simulink model "MIL_pController"  (R2018b)
settings: Solver=FixedStepAuto  StartTime=0.0  StopTime=150  FixedStep=0.001  MaxStep=0.001  RelTol=1e-3
values from neighbouring files (symbols this model uses):
  nCyclePerMinuteRef = 25    [MIL_pController_init.m]
  Pblower_tgt = 55    [MIL_pController_init.m]
  pBlowerValveOutletMaxStaticTargetRef = 200    [MIL_pController_init.m]
  pPatientValveInletTargetRef = 100    [MIL_pController_init.m]
  rInhalationPerCycleRef = 1/3    (= 0.333333333333)    [MIL_pController_init.m]
undefined symbols (not defined in the file or in its folder): BTClockRemoval, Cpoumon, Dinttuy, e, hlibtuy, Patm, Rex, Rpoumon, sigbuilder_block, tinsp, tperiod, X_makair, Y_makair
libraries: simulink x11, simulink_extras x1
settings Model: Creator=FASSI  LastModifiedBy=VITIE
settings SolverCC: AlgebraicLoopSolver=LineSearch

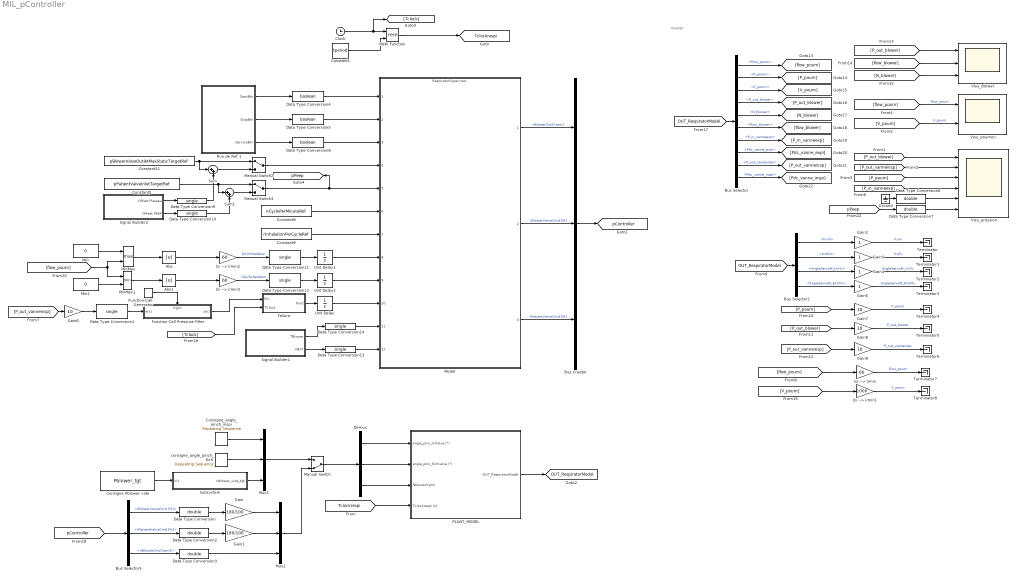
== system MIL_pController ==
  note: Viewer
  Abs : Abs
  Abs1 : Abs
  Bus Creator : BusCreator  Inputs=3
  Bus Selector : BusSelector  OutputSignals=flow_poum,P_poum,V_poum,P_out_blower,N_blower,flow_blower,P_in_vanneexp,Pdc_vanne_expi,P_out_vanneinsp,Pdc_vanne_inspi
  Bus Selector1 : BusSelector  OutputSignals=KvIn,KvExh,AngleServoM_InVlv,AngleServoM_ExhVlv
  Bus Selector5 : BusSelector  OutputSignals=rBlowerValveCmd [%],rPatientValveCmd [%],nBlowerCmd [rpm]
  Clock : Clock
  Consigne Pblower vide : Constant  Value=Pblower_tgt
  Consigne_angle_pinch_inspi : simulink/Sources/Repeating Sequence  rep_seq_t=X_insp2  rep_seq_y=[0 180 180 180 0 0 0]
  Constant1 : Constant  Value=tperiod
  Constant11 : Constant  Value=pBlowerValveOutletMaxStaticTargetRef  OutDataTypeStr=single
  Constant5 : Constant  Value=pPatientValveInletTargetRef  OutDataTypeStr=single
  Constant8 : Constant  Value=nCyclePerMinuteRef  OutDataTypeStr=single
  Constant9 : Constant  Value=rInhalationPerCycleRef  OutDataTypeStr=single
  Data Type Conversion{,2..3,6..7} (5 alike) : DataTypeConversion  OutDataTypeStr=double
  Data Type Conversion{1,9..14} (7 alike) : DataTypeConversion  OutDataTypeStr=single
  Data Type Conversion4 : DataTypeConversion  OutDataTypeStr=boolean
  Data Type Conversion5 : DataTypeConversion  OutDataTypeStr=boolean
  Data Type Conversion8 : DataTypeConversion  OutDataTypeStr=boolean
  Demux : Demux  Outputs=3
  Failure : Subsystem
  Function-Call Generator : simulink/Ports & Subsystems/Function-Call Generator  sample_time=0.005  numberOfIterations=1
  Function-Call Pressure Filter : Subsystem  TreatAsAtomicUnit=on
  Gain : Gain  Gain=180/100
  Gain1 : Gain  Gain=180/100
  Gain{2..5} (4 alike) : Gain
  Gain{6..9} (4 alike) : Gain  Gain=10
  Ground : Ground
  Manual Switch : ManualSwitch  CurrentSetting=0
  Manual Switch2 : ManualSwitch
  Manual Switch3 : ManualSwitch
  Math Function : Math  Operator=rem  SaturateOnIntegerOverflow=on
  Min : Constant  Value=0
  Min1 : Constant  Value=0
  MinMax : MinMax  Function=max  Inputs=2
  MinMax1 : MinMax  Inputs=2
  Model : ModelReference  ModelNameDialog=RespiratorSupervisor.slx  SimulationMode=Normal  ModelReferenceVersion=1.366
  Mux1 : Mux  Inputs=3
  Mux2 : Mux  Inputs=3
  PLANT_MODEL : Subsystem
  Run de Ref 1 : Subsystem  Tag=STV Subsys  LoadFcn=sigbuilder_block('load');  StartFcn=sigbuilder_block('start');  StopFcn=sigbuilder_block('stop');  ClipboardFcn=sigbuilder_block('clipboard');  mask(Sigbuilder block){tuvar=[0:10]}
      mask help: Simulink:masks:SigbuilderBlock_MD
      mask init:
      | if ~strcmp(get_param(bdroot(gcbh),'SimulationStatus'),'stopped') tuvar = sigbuilder_block('maskInit'); end
      settings: CopyFcn=sigbuilder_block('copy');  DeleteFcn=sigbuilder_block('delete');  ModelCloseFcn=sigbuilder_block('modelClose');  PreSaveFcn=sigbuilder_block('preSave');  PauseFcn=sigbuilder_block('pause');  ContinueFcn=sigbuilder_block('continue');  NameChangeFcn=sigbuilder_block('namechange');  OpenFcn=sigbuilder_block('open',[5.4 33 1141.2 514.8 ]);  CloseFcn=sigbuilder_block('close');
      mask Display: plot(0, 0, 100, 100,[2, 2, 32, 32, 2], [68, 8, 8, 68, 68],[32, 2], [38, 38], [32, 19, 2],[53, 60, 44], [32, 17, 17, 2],[16, 16, 31, 31]);txt = getActiveGroup(gcbh);text(2, 100, txt,'verticalAlignment', 'top');
  Signal Builder1 : Subsystem  Tag=STV Subsys  LoadFcn=sigbuilder_block('load');  StartFcn=sigbuilder_block('start');  StopFcn=sigbuilder_block('stop');  ClipboardFcn=sigbuilder_block('clipboard');  mask(Sigbuilder block){tuvar=[0:10]}
      mask help: Simulink:masks:SigbuilderBlock_MD
      mask init:
      | if ~strcmp(get_param(bdroot(gcbh),'SimulationStatus'),'stopped') tuvar = sigbuilder_block('maskInit'); end
      settings: CopyFcn=sigbuilder_block('copy');  DeleteFcn=sigbuilder_block('delete');  ModelCloseFcn=sigbuilder_block('modelClose');  PreSaveFcn=sigbuilder_block('preSave');  PauseFcn=sigbuilder_block('pause');  ContinueFcn=sigbuilder_block('continue');  NameChangeFcn=sigbuilder_block('namechange');  OpenFcn=sigbuilder_block('open',[5.4 30 1141.2 522.6 ]);  CloseFcn=sigbuilder_block('close');
      mask Display: plot(0, 0, 100, 100,[2, 2, 32, 32, 2], [68, 8, 8, 68, 68],[32, 2], [38, 38], [32, 19, 2],[53, 60, 44], [32, 17, 17, 2],[16, 16, 31, 31]);txt = getActiveGroup(gcbh);text(2, 100, txt,'verticalAlignment', 'top');
  Signal Builder2 : Subsystem  Tag=STV Subsys  LoadFcn=sigbuilder_block('load');  StartFcn=sigbuilder_block('start');  StopFcn=sigbuilder_block('stop');  ClipboardFcn=sigbuilder_block('clipboard');  mask(Sigbuilder block){tuvar=[0:10]}
      mask help: Simulink:masks:SigbuilderBlock_MD
      mask init:
      | if ~strcmp(get_param(bdroot(gcbh),'SimulationStatus'),'stopped') tuvar = sigbuilder_block('maskInit'); end
      settings: CopyFcn=sigbuilder_block('copy');  DeleteFcn=sigbuilder_block('delete');  ModelCloseFcn=sigbuilder_block('modelClose');  PreSaveFcn=sigbuilder_block('preSave');  PauseFcn=sigbuilder_block('pause');  ContinueFcn=sigbuilder_block('continue');  NameChangeFcn=sigbuilder_block('namechange');  OpenFcn=sigbuilder_block('open',[0 30 1152 561.6 ]);  CloseFcn=sigbuilder_block('close');
      mask Display: plot(0, 0, 100, 100,[2, 2, 32, 32, 2], [68, 8, 8, 68, 68],[32, 2], [38, 38], [32, 19, 2],[53, 60, 44], [32, 17, 17, 2],[16, 16, 31, 31]);txt = getActiveGroup(gcbh);text(2, 100, txt,'verticalAlignment', 'top');
  Subsystem : Subsystem
  Sum : Sum  Inputs=|++
  Sum1 : Sum  Inputs=|++
  Terminator{,1..8} (9 alike) : Terminator
  Unit Delay : UnitDelay  SampleTime=-1
  Unit Delay1 : UnitDelay  SampleTime=-1
  Unit Delay2 : UnitDelay  SampleTime=-1
  VIsu_Blower : Scope  NumInputPorts=3
  VIsu_poumon : Scope  NumInputPorts=2
  Visu_pression : Scope  NumInputPorts=6
  consigne_angle_pinch_Exh : simulink/Sources/Repeating Sequence  rep_seq_t=X_exp2  rep_seq_y=[0 0 0 180 180 0 0]
  l/s --> l/min : Gain  Gain=60
  l/s --> l/min1 : Gain  Gain=1000
  l/s --> l/min2 : Gain  Gain=60
  l/s --> l/min3 : Gain  Gain=60
  tag scope: OUT_RespiratorModel=global, Tclockrespi=global, pController=global, pPeep=global
  wires:
  Clock/1 -> [Tclock], Math Function/1
  Constant1/1 -> Math Function/2
  [flow_poum] -> VIsu_poumon/1  "flow_poum"
  [V_poum] -> VIsu_poumon/2  "V_poum"
  [flow_blower] -> VIsu_Blower/2
  [P_out_blower] -> VIsu_Blower/1
  [N_blower] -> VIsu_Blower/3
  Bus Selector/10 -> [Pdc_vanne_inspi]  "<Pdc_vanne_inspi>"
  Bus Selector/9 -> [P_out_vanneinsp]  "<P_out_vanneinsp>"
  Bus Selector/8 -> [Pdc_vanne_expi]  "<Pdc_vanne_expi>"
  Bus Selector/7 -> [P_in_vanneexp]  "<P_in_vanneexp>"
  Bus Selector/6 -> [flow_blower]  "<flow_blower>"
  Bus Selector/5 -> [N_blower]  "<N_blower>"
  Bus Selector/4 -> [P_out_blower]  "<P_out_blower>"
  Bus Selector/3 -> [V_poum]  "<V_poum>"
  Bus Selector/2 -> [P_poum]  "<P_poum>"
  Bus Selector/1 -> [flow_poum]  "<flow_poum>"
  [P_out_vanneinsp] -> Gain6/1
  Consigne Pblower vide/1 -> Subsystem/1(In1)
  [Tclockrespi] -> PLANT_MODEL/4(Tclockrespi (s))
  Model/3 -> Bus Creator/3  "rPatientValveCmd [%]"
  Bus Creator/1 -> [pController]
  Subsystem/1(Nblower_vide_tgt) -> Mux1/3
  consigne_angle_pinch_Exh/1 -> Mux1/2
  Consigne_angle_pinch_inspi/1 -> Mux1/1
  Demux/3 -> PLANT_MODEL/3(Nblower(rpm))
  Gain/1 -> Mux2/1
  Gain1/1 -> Mux2/2
  Bus Selector5/3 -> Data Type Conversion3/1  "<nBlowerCmd [rpm]>"
  [OUT_RespiratorModel] -> Bus Selector/1
  Model/2 -> Bus Creator/2  "rBlowerValveCmd [%]"
  Model/1 -> Bus Creator/1  "nBlowerCmd [rpm]"
  Demux/2 -> PLANT_MODEL/2(angle_pinc_Exhvalve (°))
  Demux/1 -> PLANT_MODEL/1(angle_pinc_InValve (°))
  PLANT_MODEL/1(OUT_RespiratorModel) -> [OUT_RespiratorModel]
  Math Function/1 -> [Tclockrespi]
  [P_out_blower] -> Visu_pression/1
  [P_out_vanneinsp] -> Visu_pression/2
  [P_poum] -> Visu_pression/3
  [P_in_vanneexp] -> Visu_pression/4
  Manual Switch/1 -> Demux/1
  Mux1/1 -> Manual Switch/1
  Mux2/1 -> Manual Switch/2
  Bus Selector5/1 -> Data Type Conversion/1  "<rBlowerValveCmd [%]>"
  Data Type Conversion2/1 -> Gain1/1
  Data Type Conversion/1 -> Gain/1
  Bus Selector5/2 -> Data Type Conversion2/1  "<rPatientValveCmd [%]>"
  Data Type Conversion3/1 -> Mux2/3
  [pController] -> Bus Selector5/1
  Ground/1 -> Data Type Conversion6/1
  [pPeep] -> Data Type Conversion7/1
  Data Type Conversion6/1 -> Visu_pression/5
  Data Type Conversion7/1 -> Visu_pression/6
  Gain6/1 -> Data Type Conversion1/1
  Constant11/1 -> Manual Switch2/1, Sum/1
  [OUT_RespiratorModel] -> Bus Selector1/1
  Gain5/1 -> Terminator3/1  "AngleServoM_ExhVlv"
  Gain2/1 -> Terminator/1  "KvIn"
  Bus Selector1/3 -> Gain4/1  "<AngleServoM_InVlv>"
  [P_out_blower] -> Gain8/1
  [P_out_vanneinsp] -> Gain9/1
  Gain9/1 -> Terminator6/1  "P_out_vanneinsp"
  Gain8/1 -> Terminator5/1  "P_out_blower"
  Bus Selector1/1 -> Gain2/1  "<KvIn>"
  Gain4/1 -> Terminator2/1  "AngleServoM_InVlv"
  Gain3/1 -> Terminator1/1  "KvEx"
  Bus Selector1/2 -> Gain3/1  "<KvExh>"
  Gain7/1 -> Terminator4/1  "P_poum"
  l/s --> l/min/1 -> Terminator7/1  "flow_poum"
  [flow_poum] -> l/s --> l/min/1
  Bus Selector1/4 -> Gain5/1  "<AngleServoM_ExhVlv>"
  [V_poum] -> l/s --> l/min1/1
  l/s --> l/min1/1 -> Terminator8/1  "V_poum"
  [P_poum] -> Gain7/1
  Function-Call Pressure Filter/1(y(k)) -> Failure/1(Pin)
  Data Type Conversion1/1 -> Function-Call Pressure Filter/1(e(k))
  Function-Call Generator/1 -> Function-Call Pressure Filter/Trigger
  Constant9/1 -> Model/7
  Constant8/1 -> Model/6
  Manual Switch3/1 -> [pPeep], Model/5
  Manual Switch2/1 -> Model/4
  Data Type Conversion4/1 -> Model/1
  Data Type Conversion5/1 -> Model/2
  Data Type Conversion8/1 -> Model/3
  Failure/1(Pout) -> Unit Delay/1
  [Tclock] -> Failure/2(TClock)
  Run de Ref 1/1(StartBtn) -> Data Type Conversion4/1
  Run de Ref 1/2(StopBtn) -> Data Type Conversion5/1
  Run de Ref 1/3(ServiceBtn) -> Data Type Conversion8/1
  Constant5/1 -> Sum1/1, Manual Switch3/1
  Sum/1 -> Manual Switch2/2
  Sum1/1 -> Manual Switch3/2
  Signal Builder2/1(Offset Plateau) -> Data Type Conversion9/1
  Signal Builder2/2(Offset PEEP) -> Data Type Conversion10/1
  Data Type Conversion9/1 -> Sum/2
  Data Type Conversion10/1 -> Sum1/2
  Min/1 -> MinMax/1
  [flow_poum] -> MinMax1/1, MinMax/2
  Min1/1 -> MinMax1/2
  MinMax/1 -> Abs/1
  MinMax1/1 -> Abs1/1
  Abs/1 -> l/s --> l/min2/1
  Abs1/1 -> l/s --> l/min3/1
  l/s --> l/min2/1 -> Data Type Conversion11/1  "QAirInhalation"
  l/s --> l/min3/1 -> Data Type Conversion12/1  "QAirExhalation"
  Data Type Conversion11/1 -> Unit Delay1/1
  Data Type Conversion12/1 -> Unit Delay2/1
  Unit Delay1/1 -> Model/8
  Unit Delay2/1 -> Model/9
  Unit Delay/1 -> Model/10
  Signal Builder1/1(TBlower) -> Data Type Conversion14/1
  Signal Builder1/2(VBAT) -> Data Type Conversion13/1
  Data Type Conversion13/1 -> Model/12
  Data Type Conversion14/1 -> Model/11

== system MIL_pController/Failure ==
  Pin : Inport
  TClock : Inport  Port=2
  Constant3 : Constant  Value=0  OutDataTypeStr=single
  Display : Display
  Manual Switch3 : ManualSwitch  CurrentSetting=0
  Switch1 : Switch  Threshold=25
  Pout : Outport
  wires:
  Manual Switch3/1 -> Display/1, Pout/1
  TClock/1 -> Switch1/2
  Constant3/1 -> Switch1/1
  Switch1/1 -> Manual Switch3/1
  Pin/1 -> Manual Switch3/2, Switch1/3

== system MIL_pController/Function-Call Pressure Filter ==
  e(k) : Inport
  function : TriggerPort  TriggerType=function-call  VariantControl=Variant
  Constant : Constant  Value=1/5  OutDataTypeStr=single
  Product : Product
  Sum : Sum  Inputs=|+-
  Sum1 : Sum  Inputs=|++
  Unit Delay : UnitDelay  SampleTime=-1
  y(k) : Outport
  wires:
  e(k)/1 -> Sum/1
  Unit Delay/1 -> Sum1/2, Sum/2
  Sum/1 -> Product/2
  Constant/1 -> Product/1
  Product/1 -> Sum1/1
  Sum1/1 -> y(k)/1, Unit Delay/1

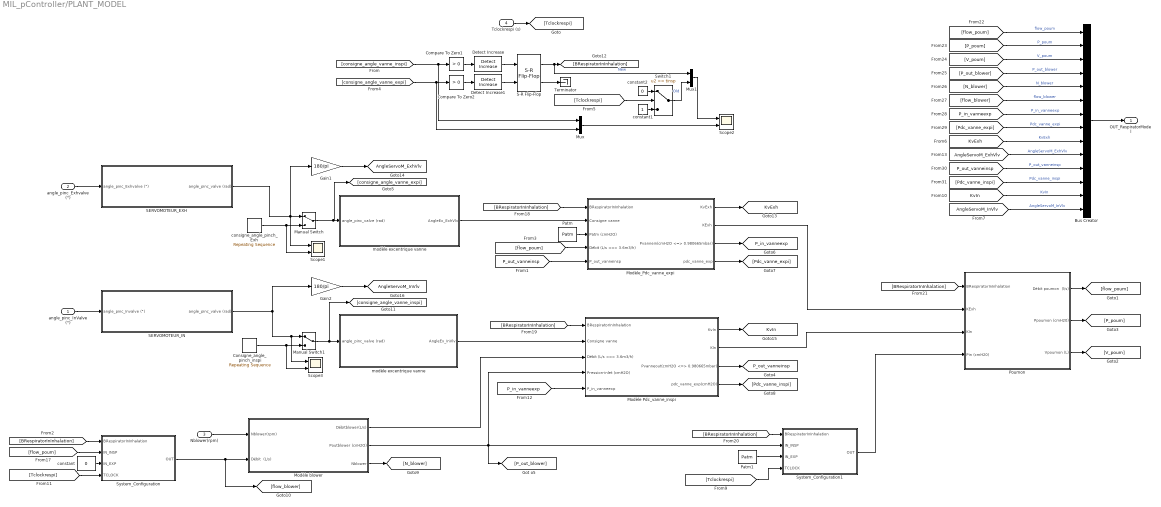
== system MIL_pController/PLANT_MODEL ==
  angle_pinc_InValve (°) : Inport
  angle_pinc_Exhvalve (°) : Inport  Port=2
  Nblower(rpm) : Inport  Port=3
  Tclockrespi (s) : Inport  Port=4
  Bus Creator : BusCreator  Inputs=14
  Compare To Zero1 : simulink/Logic and Bit Operations/Compare To Zero  relop=>  OutDataTypeStr=boolean
  Compare To Zero2 : simulink/Logic and Bit Operations/Compare To Zero  relop=>  OutDataTypeStr=boolean
  Consigne_angle_pinch_inspi : simulink/Sources/Repeating Sequence  rep_seq_t=X_insp  rep_seq_y=[0 pi pi pi 0 0 0]
  Detect Increase : simulink/Logic and Bit Operations/Detect Increase  vinit=0.0  OutDataTypeStr=boolean
  Detect Increase1 : simulink/Logic and Bit Operations/Detect Increase  vinit=0.0  OutDataTypeStr=boolean
  Gain1 : Gain  Gain=180/pi
  Gain2 : Gain  Gain=180/pi
  Manual Switch : ManualSwitch
  Manual Switch1 : ManualSwitch
  Modèle Pdc_vanne_inspi : Subsystem
  Modèle blower : Subsystem
  Modèle_Pdc_vanne_expi : Subsystem
  Mux : Mux  Inputs=2
  Mux1 : Mux  Inputs=2
  Patm : Constant  Value=Patm
  Patm1 : Constant  Value=Patm
  Poumon : Subsystem
  S-R Flip-Flop : simulink_extras/Flip Flops/S-R Flip-Flop  initial_condition=1
  SERVOMOTEUR_EXH : Subsystem
  SERVOMOTEUR_IN : Subsystem
  Scope1 : Scope  NumInputPorts=2
  Scope2 : Scope  NumInputPorts=2
  Scope3 : Scope  NumInputPorts=2
  Switch1 : Switch  Threshold=tinsp
  System_Configuration : Subsystem
  System_Configuration1 : Subsystem
  Terminator : Terminator
  consigne_angle_pinch_Exh : simulink/Sources/Repeating Sequence  rep_seq_t=X_exp  rep_seq_y=[0 0 0 pi pi 0 0]
  constant : Constant  Value=0
  constant1 : Constant  OutDataTypeStr=boolean
  constant2 : Constant  Value=0  OutDataTypeStr=boolean
  modèle excentrique vanne : Subsystem
  "modèle excentrique vanne " : Subsystem
  OUT_RespiratorModel : Outport
  tag scope: AngleServoM_ExhVlv=global, AngleServoM_InVlv=global, KvExh=global, KvIn=global, P_in_vanneexp=global, P_out_vanneinsp=global
  wires:
  Modèle Pdc_vanne_inspi/1(KvIn) -> [KvIn]
  Modèle_Pdc_vanne_expi/1(KvExh) -> [KvExh]
  Gain2/1 -> [AngleServoM_InVlv]
  Gain1/1 -> [AngleServoM_ExhVlv]
  consigne_angle_pinch_Exh/1 -> Manual Switch/2, Scope1/2
  [KvIn] -> Bus Creator/13  "KvIn"
  [AngleServoM_InVlv] -> Bus Creator/14  "AngleServoM_InVlv"
  [AngleServoM_ExhVlv] -> Bus Creator/10  "AngleServoM_ExhVlv"
  [KvExh] -> Bus Creator/9  "KvExh"
  Manual Switch1/1 -> "modèle excentrique vanne "/1(angle_pinc_valve (rad)), [consigne_angle_vanne_inspi]
  Consigne_angle_pinch_inspi/1 -> Manual Switch1/2, Scope3/2
  angle_pinc_InValve (°)/1 -> SERVOMOTEUR_IN/1(angle_pinc_Invalve (°))
  SERVOMOTEUR_IN/1(angle_pinc_valve (rad)) -> Gain2/1, Manual Switch1/1, Scope3/1
  Manual Switch/1 -> modèle excentrique vanne/1(angle_pinc_valve (rad)), [consigne_angle_vanne_expi]
  SERVOMOTEUR_EXH/1(angle_pinc_valve (rad)) -> Manual Switch/1, Gain1/1, Scope1/1
  angle_pinc_Exhvalve (°)/1 -> SERVOMOTEUR_EXH/1(angle_pinc_Exhvalve (°))
  constant2/1 -> Switch1/1
  constant1/1 -> Switch1/3
  Mux1/1 -> Scope2/1
  Switch1/1 -> Mux1/2  "Old"
  [Tclockrespi] -> Switch1/2
  Mux/1 -> Scope2/2
  Tclockrespi (s)/1 -> [Tclockrespi]
  Nblower(rpm)/1 -> Modèle blower/1(Nblower(rpm))
  [P_poum] -> Bus Creator/2  "P_poum"
  [Pdc_vanne_expi] -> Bus Creator/8  "Pdc_vanne_expi"
  [P_in_vanneexp] -> Bus Creator/7  "P_in_vanneexp"
  [P_out_blower] -> Bus Creator/4  "P_out_blower"
  Modèle blower/3(Nblower) -> [N_blower]
  Modèle Pdc_vanne_inspi/3(Pvanneout(cmH2O <=> 0.980665mbar)) -> [P_out_vanneinsp]
  Modèle_Pdc_vanne_expi/3(Pvannein(cmH2O <=> 0.980665mbar)) -> [P_in_vanneexp]
  Modèle Pdc_vanne_inspi/4(pdc_vanne_exp(cmH2O)) -> [Pdc_vanne_inspi]
  Modèle Pdc_vanne_inspi/2(KIn) -> Poumon/3("KIn ")
  [N_blower] -> Bus Creator/5  "N_blower"
  [BRespiratorInInhalation] -> Modèle Pdc_vanne_inspi/1(BRespiratorInInhalation)
  modèle excentrique vanne/1(AngleEx_ExhVlv) -> Modèle_Pdc_vanne_expi/2(Consigne vanne)
  [flow_poum] -> Modèle_Pdc_vanne_expi/4(Débit (L/s <=> 3.6m3/h))
  [Tclockrespi] -> System_Configuration1/4(TCLOCK)
  Modèle blower/1(Débitblower(L/s)) -> Modèle Pdc_vanne_inspi/3(Débit (L/s <=> 3.6m3/h))
  Poumon/2(Ppoumon (cmH20)) -> [P_poum]
  Detect Increase/1 -> S-R Flip-Flop/1
  [P_out_vanneinsp] -> Bus Creator/11  "P_out_vanneinsp"
  [flow_poum] -> System_Configuration/2(IN_INSP)
  [P_out_vanneinsp] -> Modèle_Pdc_vanne_expi/5(P_out_vanneinsp)
  [flow_blower] -> Bus Creator/6  "flow_blower"
  [flow_poum] -> Bus Creator/1  "flow_poum"
  Bus Creator/1 -> OUT_RespiratorModel/1
  [consigne_angle_vanne_inspi] -> Compare To Zero1/1, Mux/1
  Modèle blower/2(Poutblower (cnH2O)) -> Modèle Pdc_vanne_inspi/4(Pression-inlet (cmH2O)), System_Configuration1/2(IN_INSP), [P_out_blower]
  S-R Flip-Flop/2 -> Terminator/1
  [Tclockrespi] -> System_Configuration/4(TCLOCK)
  "modèle excentrique vanne "/1(AngleEx_InVlv) -> Modèle Pdc_vanne_inspi/2(Consigne vanne)
  Detect Increase1/1 -> S-R Flip-Flop/2
  Poumon/1(Débit poumon  (l/s)) -> [flow_poum]
  Poumon/3(Vpoumon (L)) -> [V_poum]
  Patm1/1 -> System_Configuration1/3(IN_EXP)
  constant/1 -> System_Configuration/3(IN_EXP)
  [consigne_angle_vanne_expi] -> Compare To Zero2/1, Mux/2
  [Pdc_vanne_inspi] -> Bus Creator/12  "Pdc_vanne_inspi"
  Modèle_Pdc_vanne_expi/4(pdc_vanne_exp) -> [Pdc_vanne_expi]
  [BRespiratorInInhalation] -> Modèle_Pdc_vanne_expi/1(BRespiratorInInhalation)
  [BRespiratorInInhalation] -> Poumon/1(BRespiratorInInhalation)
  System_Configuration1/1(OUT) -> Poumon/4(Pin (cmH20))
  S-R Flip-Flop/1 -> [BRespiratorInInhalation], Mux1/1  "New"
  [BRespiratorInInhalation] -> System_Configuration/1(BRespiratorInInhalation)
  Compare To Zero2/1 -> Detect Increase1/1
  [P_in_vanneexp] -> Modèle Pdc_vanne_inspi/5(P_in_vanneexp)
  [BRespiratorInInhalation] -> System_Configuration1/1(BRespiratorInInhalation)
  Patm/1 -> Modèle_Pdc_vanne_expi/3(Patm (cmH2O))
  System_Configuration/1(OUT) -> Modèle blower/2(Débit  (L/s)), [flow_blower]
  Modèle_Pdc_vanne_expi/2(KExh) -> Poumon/2(KExh)
  Compare To Zero1/1 -> Detect Increase/1
  [V_poum] -> Bus Creator/3  "V_poum"

== system MIL_pController/Run de Ref 1 ==
  Demux : Demux  Tag=STV Demux  Outputs=3
  FromWs : FromWorkspace  Tag=STV FromWs  VariableName=tuvar  SampleTime=0
      SigBuilderData=|
      | common.afterFinalStr = 'Extrapolate'
      | common.sampleTime = 0
      | dataSet.timeRange = [0 100]
      | dataSet.name = 'Group 1'
      | sbobj.Groups.Name = 'Group 1'
      | sbobj.Groups.Signals(1).Name = 'StartBtn'
      | sbobj.Groups.Signals(1).XData = [0 0.5 1.5 2 2.5 3 3 3.4 3.4 9.2 9.2 9.7 9.7 14.6 14.6 15.2 15.2 59.5 59.5 60 60 100]
      | sbobj.Groups.Signals(1).YData = [0 0 0 0 0 0 1 1 0 0 1 1 0 0 1 1 0 0 1 1 0 0]
      | sbobj.Groups.Signals(2).Name = 'StopBtn'
      | sbobj.Groups.Signals(2).XData = [0 5 5 10 15 24.6 24.6 25 25 34.6 34.6 35 35 48.7 48.7 49.2 49.2 50 50 50.5 50.5 64.7 64.7 65 65 74.7 74.7 75 75 87.6 87.6 88 88 89.3 89.3 89.7 89.7 100]
      | sbobj.Groups.Signals(2).YData = [2 2 0 0 0 0 2 2 0 0 2 2 0 0 2 2 0 0 2 2 0 0 2 2 0 0 2 2 0 0 2 2 0 0 2 2 0 0]
      | sbobj.Groups.Signals(3).Name = 'ServiceBtn'
      | sbobj.Groups.Signals(3).XData = [0 0.43 0.43 1.5 1.5 7.3 7.3 11.3 13.94 100]
      | sbobj.Groups.Signals(3).YData = [1 1 0 0 1 1 0 0 0 0]
      | sbobj.Groups.TimeRange = [0 100]
  StartBtn : Outport  Tag=STV Outport
  StopBtn : Outport  Tag=STV Outport  Port=2
  ServiceBtn : Outport  Tag=STV Outport  Port=3
  wires:
  FromWs/1 -> Demux/1
  Demux/1 -> StartBtn/1
  Demux/2 -> StopBtn/1
  Demux/3 -> ServiceBtn/1

== system MIL_pController/Signal Builder1 ==
  Demux : Demux  Tag=STV Demux  Outputs=2
  FromWs : FromWorkspace  Tag=STV FromWs  VariableName=tuvar  SampleTime=0
      SigBuilderData=|
      | common.afterFinalStr = 'Extrapolate'
      | common.sampleTime = 0
      | dataSet.timeRange = [0 150]
      | dataSet.name = 'Group 1'
      | sbobj.Groups.Name = 'Group 1'
      | sbobj.Groups.Signals(1).Name = 'TBlower'
      | sbobj.Groups.Signals(1).XData = [0 5 5 10 10 30.2 30.2 70 70 110 110 130 130 150]
      | sbobj.Groups.Signals(1).YData = [20 20 48.5 48.5 19.5 19.5 84 84 39 39 78 78 20 20]
      | sbobj.Groups.Signals(2).Name = 'VBAT'
      | sbobj.Groups.Signals(2).XData = [0 50 50 90 90 95 95 150]
      | sbobj.Groups.Signals(2).YData = [48 48 26.6 26.6 23 23 25 25]
      | sbobj.Groups.TimeRange = [0 150]
  TBlower : Outport  Tag=STV Outport
  VBAT : Outport  Tag=STV Outport  Port=2
  wires:
  FromWs/1 -> Demux/1
  Demux/1 -> TBlower/1
  Demux/2 -> VBAT/1

== system MIL_pController/Signal Builder2 ==
  Demux : Demux  Tag=STV Demux  Outputs=2
  FromWs : FromWorkspace  Tag=STV FromWs  VariableName=tuvar  SampleTime=0
      SigBuilderData=|
      | common.afterFinalStr = 'Extrapolate'
      | common.sampleTime = 0
      | dataSet.timeRange = [0 150]
      | dataSet.name = 'Group 1'
      | sbobj.Groups.Name = 'Group 1'
      | sbobj.Groups.Signals(1).Name = 'Offset Plateau'
      | sbobj.Groups.Signals(1).XData = [0 5 10 30.2 30.2 70 70 110 110 130 130 150]
      | sbobj.Groups.Signals(1).YData = [-50 -50 -50 -50 49.8 49.8 0 0 50 50 -45 -45]
      | sbobj.Groups.Signals(2).Name = 'Offset PEEP'
      | sbobj.Groups.Signals(2).XData = [0 50 50 90 90 95 150]
      | sbobj.Groups.Signals(2).YData = [0 0 100 100 50 50 50]
      | sbobj.Groups.TimeRange = [0 150]
  Offset Plateau : Outport  Tag=STV Outport
  Offset PEEP : Outport  Tag=STV Outport  Port=2
  wires:
  FromWs/1 -> Demux/1
  Demux/1 -> Offset Plateau/1
  Demux/2 -> Offset PEEP/1

== system MIL_pController/Subsystem ==
  In1 : Inport
  1-D Lookup Table3 : Lookup_n-D  NumberOfTableDimensions=1  LookupTableObject=vanne_makair  BreakpointsForDimension1=[32 64 104]  Table=[30000 41000 54000]  InternalRulePriority=Speed  RndMeth=Simplest  InputSameDT=on
  Nblower_vide_tgt : Outport
  wires:
  1-D Lookup Table3/1 -> Nblower_vide_tgt/1
  In1/1 -> 1-D Lookup Table3/1

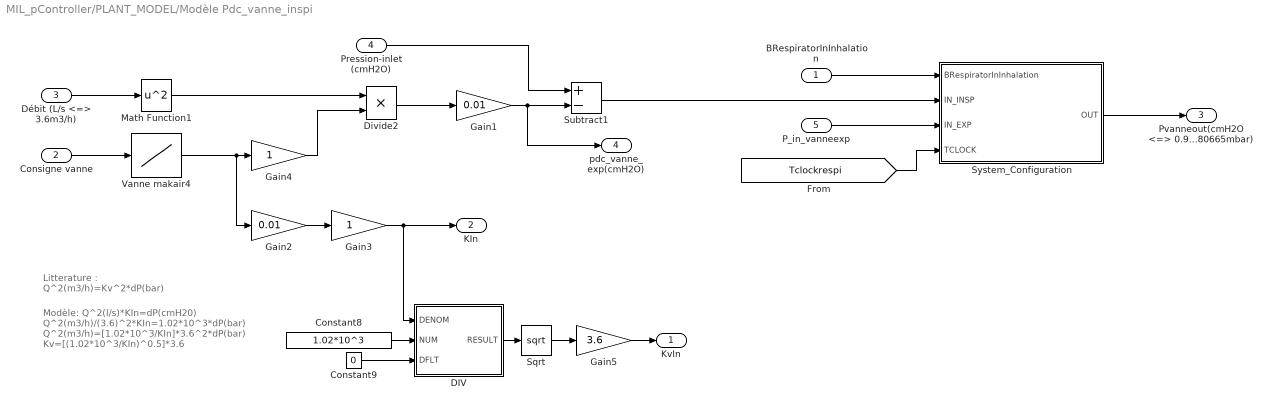
== system MIL_pController/PLANT_MODEL/Modèle Pdc_vanne_inspi ==
  note: Modèle:
      | Q^2(l/s)*KIn=dP(cmH20)
      | Q^2(m3/h)/(3.6)^2*KIn=1.02*10^3*dP(bar)
      | Q^2(m3/h)=[1.02*10^3/KIn]*3.6^2*dP(bar)
      |
      | Kv=[(1.02*10^3/KIn)^0.5]*3.6
  note: Litterature :
      | Q^2(m3/h)=Kv^2*dP(bar)
  BRespiratorInInhalation : Inport
  Consigne vanne : Inport  Port=2
  Débit (L/s <=> 3.6m3/h) : Inport  Port=3
  Pression-inlet (cmH2O) : Inport  Port=4
  P_in_vanneexp : Inport  Port=5
  Constant8 : Constant  Value=1.02*10^3
  Constant9 : Constant  Value=0
  DIV : Subsystem  mask(DIV){}
      mask help: This block executes a division with protection for division by 0.
      mask Display: disp('DIV')
  Divide2 : Product  Inputs=**
  Gain1 : Gain  Gain=0.01
  Gain2 : Gain  Gain=0.01
  Gain3 : Gain
  Gain4 : Gain
  Gain5 : Gain  Gain=3.6
  Math Function1 : Math  Operator=square  SaturateOnIntegerOverflow=on
  Sqrt : Sqrt  SaturateOnIntegerOverflow=on
  Subtract1 : Sum  Inputs=+-
  System_Configuration : Subsystem
  Vanne makair4 : Lookup_n-D  NumberOfTableDimensions=1  LookupTableObject=vanne_makair  BreakpointsForDimension1=X_makair  Table=Y_makair  InternalRulePriority=Speed  RndMeth=Simplest  InputSameDT=on
  KvIn : Outport
  KIn : Outport  Port=2
  Pvanneout(cmH2O <=> 0.980665mbar) : Outport  Port=3
  pdc_vanne_exp(cmH2O) : Outport  Port=4
  wires:
  DIV/1(RESULT) -> Sqrt/1
  Constant8/1 -> DIV/2(NUM)
  Sqrt/1 -> Gain5/1
  Gain3/1 -> KIn/1, DIV/1(DENOM)
  Constant9/1 -> DIV/3(DFLT)
  Gain5/1 -> KvIn/1
  BRespiratorInInhalation/1 -> System_Configuration/1(BRespiratorInInhalation)
  Subtract1/1 -> System_Configuration/2(IN_INSP)
  [Tclockrespi] -> System_Configuration/4(TCLOCK)
  P_in_vanneexp/1 -> System_Configuration/3(IN_EXP)
  Gain4/1 -> Divide2/2
  System_Configuration/1(OUT) -> Pvanneout(cmH2O <=> 0.980665mbar)/1
  Gain2/1 -> Gain3/1
  Gain1/1 -> Subtract1/2, pdc_vanne_exp(cmH2O)/1
  Pression-inlet (cmH2O)/1 -> Subtract1/1
  Divide2/1 -> Gain1/1
  Consigne vanne/1 -> Vanne makair4/1
  Débit (L/s <=> 3.6m3/h)/1 -> Math Function1/1
  Vanne makair4/1 -> Gain4/1, Gain2/1
  Math Function1/1 -> Divide2/1

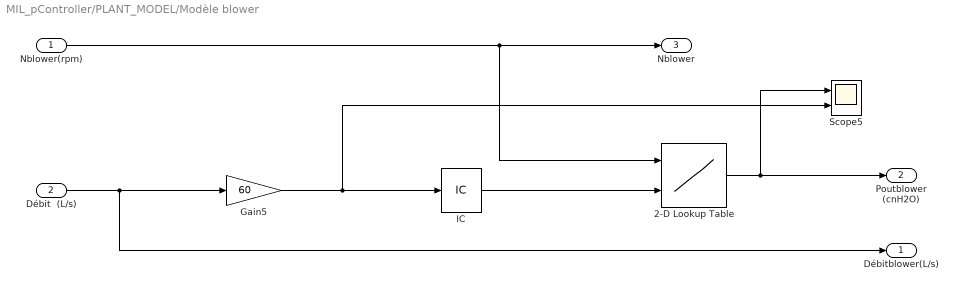
== system MIL_pController/PLANT_MODEL/Modèle blower ==
  Nblower(rpm) : Inport
  Débit  (L/s) : Inport  Port=2
  2-D Lookup Table : Lookup_n-D  BreakpointsForDimension1=[0,30000,41000,54000]  BreakpointsForDimension2=[0,15,30,50,80,100,120,140,160]  Table=reshape([0,32.2,60.6,103.8,0,31.8,59.6,103.5,0,31,59.1,102.2,0,29.2,56.5,100,0,24.8,52.4,93.7,0,20,48.2,88.8,0,15.2,43.8,82.8,0,9.1,36.3,77.2,0,1.4,29.1,71.6],4,9)  ExtrapMethod=Clip  InternalRulePriority=Speed  RndMeth=Simplest  InputSameDT=on
  Gain5 : Gain  Gain=60
  IC : InitialCondition  Value=0
  Scope5 : Scope  NumInputPorts=2
  Débitblower(L/s) : Outport
  Poutblower (cnH2O) : Outport  Port=2
  Nblower : Outport  Port=3
  wires:
  IC/1 -> 2-D Lookup Table/2
  2-D Lookup Table/1 -> Poutblower (cnH2O)/1, Scope5/1
  Débit  (L/s)/1 -> Gain5/1, Débitblower(L/s)/1
  Nblower(rpm)/1 -> Nblower/1, 2-D Lookup Table/1
  Gain5/1 -> IC/1, Scope5/2

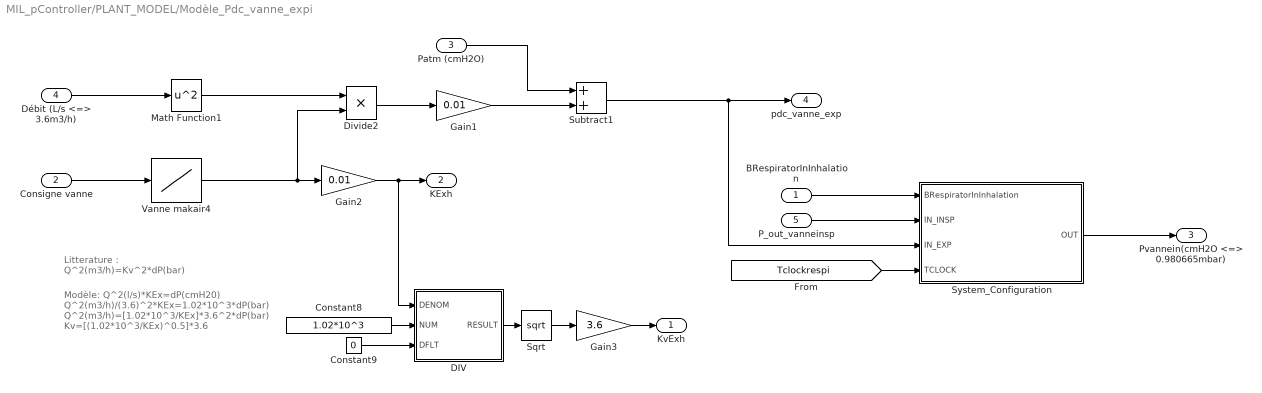
== system MIL_pController/PLANT_MODEL/Modèle_Pdc_vanne_expi ==
  note: Modèle:
      | Q^2(l/s)*KEx=dP(cmH20)
      | Q^2(m3/h)/(3.6)^2*KEx=1.02*10^3*dP(bar)
      | Q^2(m3/h)=[1.02*10^3/KEx]*3.6^2*dP(bar)
      |
      | Kv=[(1.02*10^3/KEx)^0.5]*3.6
  note: Litterature :
      | Q^2(m3/h)=Kv^2*dP(bar)
  BRespiratorInInhalation : Inport
  Consigne vanne : Inport  Port=2
  Patm (cmH2O) : Inport  Port=3
  Débit (L/s <=> 3.6m3/h) : Inport  Port=4
  P_out_vanneinsp : Inport  Port=5
  Constant8 : Constant  Value=1.02*10^3
  Constant9 : Constant  Value=0
  DIV : Subsystem  mask(DIV){}
      mask help: This block executes a division with protection for division by 0.
      mask Display: disp('DIV')
  Divide2 : Product  Inputs=**
  Gain1 : Gain  Gain=0.01
  Gain2 : Gain  Gain=0.01
  Gain3 : Gain  Gain=3.6
  Math Function1 : Math  Operator=square  SaturateOnIntegerOverflow=on
  Sqrt : Sqrt  SaturateOnIntegerOverflow=on
  Subtract1 : Sum
  System_Configuration : Subsystem
  Vanne makair4 : Lookup_n-D  NumberOfTableDimensions=1  LookupTableObject=vanne_makair  BreakpointsForDimension1=X_makair  Table=Y_makair  InternalRulePriority=Speed  RndMeth=Simplest  InputSameDT=on
  KvExh : Outport
  KExh : Outport  Port=2
  Pvannein(cmH2O <=> 0.980665mbar) : Outport  Port=3
  pdc_vanne_exp : Outport  Port=4
  wires:
  Gain3/1 -> KvExh/1
  Sqrt/1 -> Gain3/1
  DIV/1(RESULT) -> Sqrt/1
  Constant9/1 -> DIV/3(DFLT)
  Vanne makair4/1 -> Divide2/2, Gain2/1
  Constant8/1 -> DIV/2(NUM)
  P_out_vanneinsp/1 -> System_Configuration/2(IN_INSP)
  System_Configuration/1(OUT) -> Pvannein(cmH2O <=> 0.980665mbar)/1
  BRespiratorInInhalation/1 -> System_Configuration/1(BRespiratorInInhalation)
  [Tclockrespi] -> System_Configuration/4(TCLOCK)
  Subtract1/1 -> pdc_vanne_exp/1, System_Configuration/3(IN_EXP)
  Gain2/1 -> KExh/1, DIV/1(DENOM)
  Gain1/1 -> Subtract1/2
  Patm (cmH2O)/1 -> Subtract1/1
  Divide2/1 -> Gain1/1
  Consigne vanne/1 -> Vanne makair4/1
  Débit (L/s <=> 3.6m3/h)/1 -> Math Function1/1
  Math Function1/1 -> Divide2/1

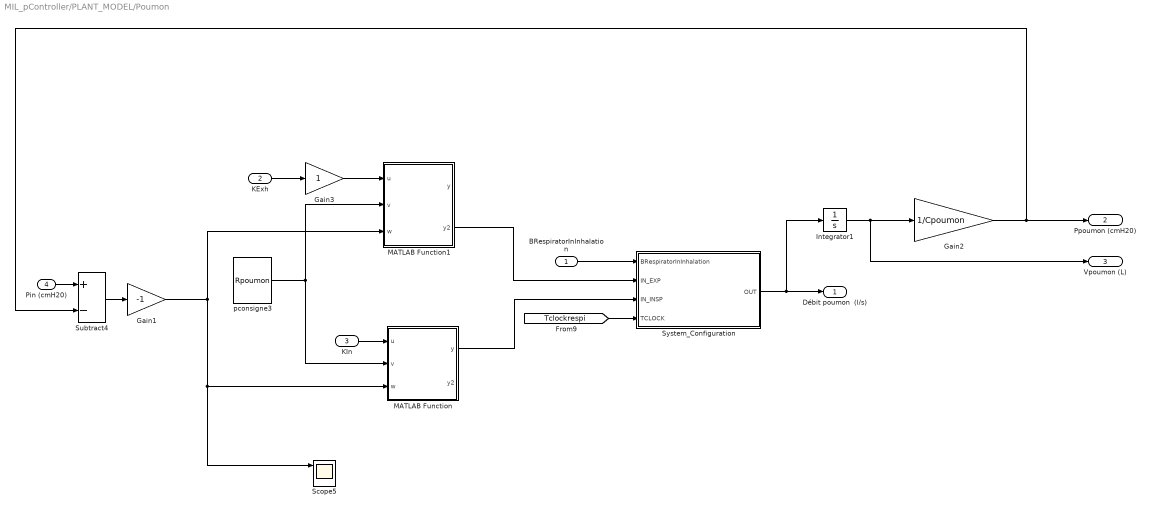
== system MIL_pController/PLANT_MODEL/Poumon ==
  BRespiratorInInhalation : Inport
  KExh : Inport  Port=2
  "KIn " : Inport  Port=3
  Pin (cmH20) : Inport  Port=4
  Gain1 : Gain  Gain=-1
  Gain2 : Gain  Gain=1/Cpoumon
  Gain3 : Gain
  Integrator1 : Integrator
  MATLAB Function : MATLAB Function  TreatAsAtomicUnit=on
  MATLAB Function1 : MATLAB Function  TreatAsAtomicUnit=on
  Scope5 : Scope  NumInputPorts=3
  Subtract4 : Sum  Inputs=+-
  System_Configuration : Subsystem
  pconsigne3 : Constant  Value=Rpoumon
  Débit poumon  (l/s) : Outport
  Ppoumon (cmH20) : Outport  Port=2
  Vpoumon (L) : Outport  Port=3
  wires:
  BRespiratorInInhalation/1 -> System_Configuration/1(BRespiratorInInhalation)
  [Tclockrespi] -> System_Configuration/4(TCLOCK)
  MATLAB Function1/2(y2) -> System_Configuration/2(IN_EXP)
  System_Configuration/1(OUT) -> Débit poumon  (l/s)/1, Integrator1/1
  Gain3/1 -> MATLAB Function1/1(u)
  KExh/1 -> Gain3/1
  Subtract4/1 -> Gain1/1
  MATLAB Function/1(y) -> System_Configuration/3(IN_INSP)
  Integrator1/1 -> Gain2/1, Vpoumon (L)/1
  "KIn "/1 -> MATLAB Function/1(u)
  Gain1/1 -> Scope5/1, MATLAB Function/3(w), MATLAB Function1/3(w)
  pconsigne3/1 -> MATLAB Function/2(v), MATLAB Function1/2(v)
  Pin (cmH20)/1 -> Subtract4/1
  Gain2/1 -> Ppoumon (cmH20)/1, Subtract4/2

== system MIL_pController/PLANT_MODEL/SERVOMOTEUR_EXH ==
  angle_pinc_Exhvalve (°) : Inport
  Gain : Gain  Gain=pi/180
  Rate Limiter Dynamic : simulink/Discontinuities/Rate Limiter Dynamic
      settings: SourceProductName=Simulink
  Slope : Constant  Value=pi/0.05
  Slope1 : Constant  Value=-pi/0.05
  angle_pinc_valve (rad) : Outport
  wires:
  Slope1/1 -> Rate Limiter Dynamic/3
  Slope/1 -> Rate Limiter Dynamic/1
  Gain/1 -> Rate Limiter Dynamic/2
  Rate Limiter Dynamic/1 -> angle_pinc_valve (rad)/1
  angle_pinc_Exhvalve (°)/1 -> Gain/1

== system MIL_pController/PLANT_MODEL/SERVOMOTEUR_IN ==
  angle_pinc_Invalve (°) : Inport
  Gain : Gain  Gain=pi/180
  Rate Limiter Dynamic : simulink/Discontinuities/Rate Limiter Dynamic
      settings: SourceProductName=Simulink
  Slope : Constant  Value=pi/0.05
  Slope1 : Constant  Value=-pi/0.05
  angle_pinc_valve (rad) : Outport
  wires:
  Gain/1 -> Rate Limiter Dynamic/2
  Slope/1 -> Rate Limiter Dynamic/1
  Slope1/1 -> Rate Limiter Dynamic/3
  angle_pinc_Invalve (°)/1 -> Gain/1
  Rate Limiter Dynamic/1 -> angle_pinc_valve (rad)/1

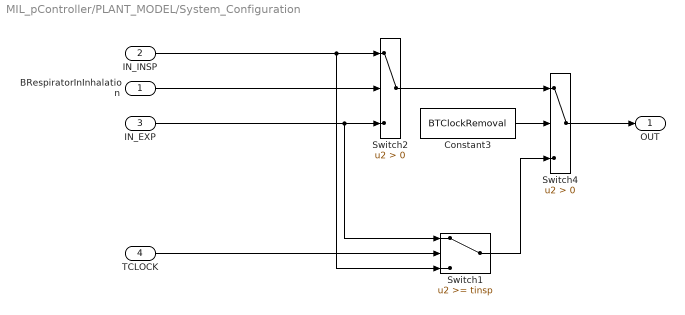
== system MIL_pController/PLANT_MODEL/System_Configuration ==
  BRespiratorInInhalation : Inport
  IN_INSP : Inport  Port=2
  IN_EXP : Inport  Port=3
  TCLOCK : Inport  Port=4
  Constant3 : Constant  Value=BTClockRemoval
  Switch1 : Switch  Threshold=tinsp
  Switch2 : Switch  Criteria=u2 > Threshold
      settings: AttributesFormatString=%<Criteria>
  Switch4 : Switch  Criteria=u2 > Threshold
      settings: AttributesFormatString=%<Criteria>
  OUT : Outport
  wires:
  IN_EXP/1 -> Switch2/3, Switch1/1
  BRespiratorInInhalation/1 -> Switch2/2
  IN_INSP/1 -> Switch2/1, Switch1/3
  Switch4/1 -> OUT/1
  TCLOCK/1 -> Switch1/2
  Switch1/1 -> Switch4/3
  Switch2/1 -> Switch4/1
  Constant3/1 -> Switch4/2

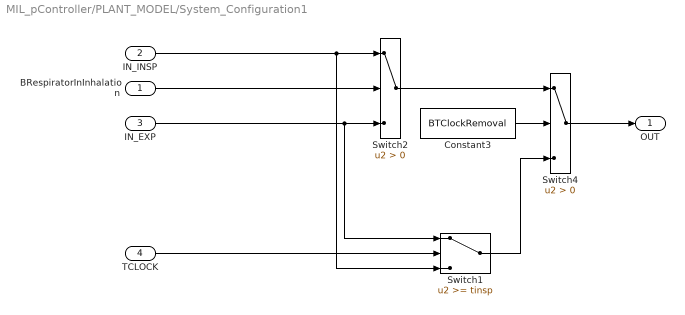
== system MIL_pController/PLANT_MODEL/System_Configuration1 ==
  BRespiratorInInhalation : Inport
  IN_INSP : Inport  Port=2
  IN_EXP : Inport  Port=3
  TCLOCK : Inport  Port=4
  Constant3 : Constant  Value=BTClockRemoval
  Switch1 : Switch  Threshold=tinsp
  Switch2 : Switch  Criteria=u2 > Threshold
      settings: AttributesFormatString=%<Criteria>
  Switch4 : Switch  Criteria=u2 > Threshold
      settings: AttributesFormatString=%<Criteria>
  OUT : Outport
  wires:
  IN_EXP/1 -> Switch2/3, Switch1/1
  BRespiratorInInhalation/1 -> Switch2/2
  IN_INSP/1 -> Switch2/1, Switch1/3
  Switch4/1 -> OUT/1
  TCLOCK/1 -> Switch1/2
  Switch1/1 -> Switch4/3
  Switch2/1 -> Switch4/1
  Constant3/1 -> Switch4/2

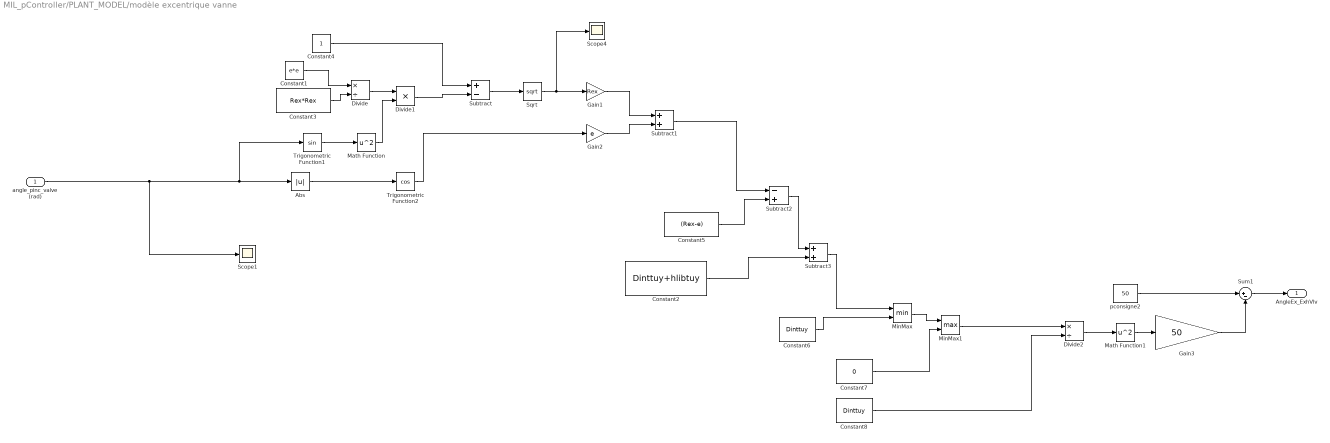
== system MIL_pController/PLANT_MODEL/modèle excentrique vanne ==
  angle_pinc_valve (rad) : Inport
  Abs : Abs
  Constant1 : Constant  Value=e*e
  Constant2 : Constant  Value=Dinttuy+hlibtuy
  Constant3 : Constant  Value=Rex*Rex
  Constant4 : Constant
  Constant5 : Constant  Value=(Rex-e)
  Constant6 : Constant  Value=Dinttuy
  Constant7 : Constant  Value=0
  Constant8 : Constant  Value=Dinttuy
  Divide : Product  Inputs=*/
  Divide1 : Product  Inputs=**
  Divide2 : Product  Inputs=*/
  Gain1 : Gain  Gain=Rex
  Gain2 : Gain  Gain=e
  Gain3 : Gain  Gain=50
  Math Function : Math  Operator=square  SaturateOnIntegerOverflow=on
  Math Function1 : Math  Operator=square  SaturateOnIntegerOverflow=on
  MinMax : MinMax  Inputs=2
  MinMax1 : MinMax  Function=max  Inputs=2
  Scope1 : Scope
  Scope4 : Scope
  Sqrt : Sqrt  SaturateOnIntegerOverflow=on
  Subtract : Sum  Inputs=+-
  Subtract1 : Sum
  Subtract2 : Sum  Inputs=-+
  Subtract3 : Sum
  Sum1 : Sum  Inputs=|+-
  Trigonometric Function1 : Trigonometry
  Trigonometric Function2 : Trigonometry  Operator=cos
  pconsigne2 : Constant  Value=50
  AngleEx_ExhVlv : Outport
  wires:
  Math Function1/1 -> Gain3/1
  pconsigne2/1 -> Sum1/1
  Gain3/1 -> Sum1/2
  Sum1/1 -> AngleEx_ExhVlv/1
  Divide2/1 -> Math Function1/1
  Constant8/1 -> Divide2/2
  MinMax1/1 -> Divide2/1
  Constant7/1 -> MinMax1/2
  MinMax/1 -> MinMax1/1
  Subtract3/1 -> MinMax/1
  Constant6/1 -> MinMax/2
  Subtract2/1 -> Subtract3/1
  Constant2/1 -> Subtract3/2
  Constant5/1 -> Subtract2/2
  Trigonometric Function2/1 -> Gain2/1
  Divide/1 -> Divide1/1
  angle_pinc_valve (rad)/1 -> Abs/1, Trigonometric Function1/1, Scope1/1
  Gain2/1 -> Subtract1/2
  Math Function/1 -> Divide1/2
  Sqrt/1 -> Gain1/1, Scope4/1
  Abs/1 -> Trigonometric Function2/1
  Gain1/1 -> Subtract1/1
  Subtract1/1 -> Subtract2/1
  Constant3/1 -> Divide/2
  Subtract/1 -> Sqrt/1
  Divide1/1 -> Subtract/2
  Constant4/1 -> Subtract/1
  Trigonometric Function1/1 -> Math Function/1
  Constant1/1 -> Divide/1

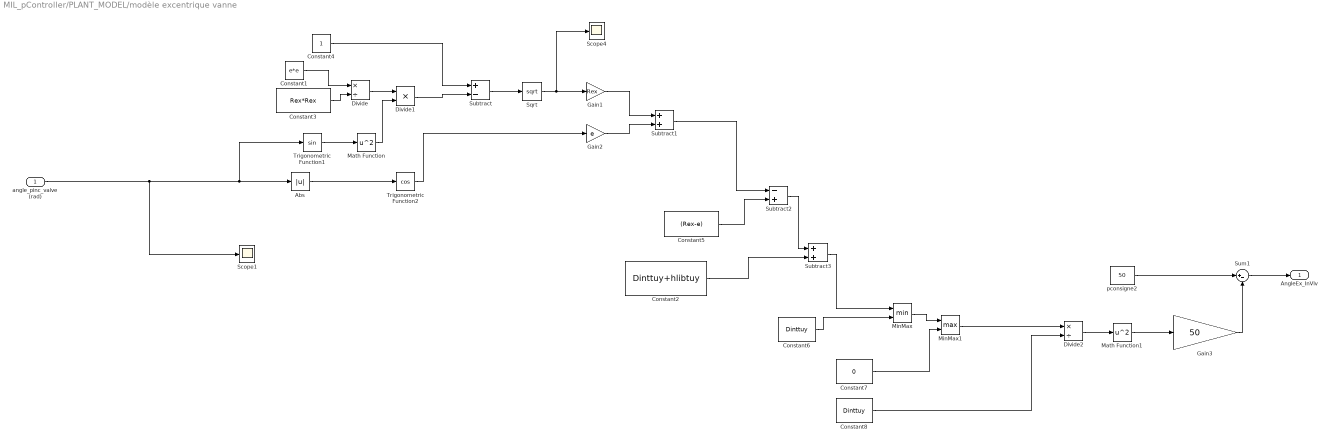
== system MIL_pController/PLANT_MODEL/modèle excentrique vanne  ==
  angle_pinc_valve (rad) : Inport
  Abs : Abs
  Constant1 : Constant  Value=e*e
  Constant2 : Constant  Value=Dinttuy+hlibtuy
  Constant3 : Constant  Value=Rex*Rex
  Constant4 : Constant
  Constant5 : Constant  Value=(Rex-e)
  Constant6 : Constant  Value=Dinttuy
  Constant7 : Constant  Value=0
  Constant8 : Constant  Value=Dinttuy
  Divide : Product  Inputs=*/
  Divide1 : Product  Inputs=**
  Divide2 : Product  Inputs=*/
  Gain1 : Gain  Gain=Rex
  Gain2 : Gain  Gain=e
  Gain3 : Gain  Gain=50
  Math Function : Math  Operator=square  SaturateOnIntegerOverflow=on
  Math Function1 : Math  Operator=square  SaturateOnIntegerOverflow=on
  MinMax : MinMax  Inputs=2
  MinMax1 : MinMax  Function=max  Inputs=2
  Scope1 : Scope
  Scope4 : Scope
  Sqrt : Sqrt  SaturateOnIntegerOverflow=on
  Subtract : Sum  Inputs=+-
  Subtract1 : Sum
  Subtract2 : Sum  Inputs=-+
  Subtract3 : Sum
  Sum1 : Sum  Inputs=|+-
  Trigonometric Function1 : Trigonometry
  Trigonometric Function2 : Trigonometry  Operator=cos
  pconsigne2 : Constant  Value=50
  AngleEx_InVlv : Outport
  wires:
  Math Function1/1 -> Gain3/1
  pconsigne2/1 -> Sum1/1
  Gain3/1 -> Sum1/2
  Sum1/1 -> AngleEx_InVlv/1
  Divide2/1 -> Math Function1/1
  Constant8/1 -> Divide2/2
  MinMax1/1 -> Divide2/1
  Constant7/1 -> MinMax1/2
  MinMax/1 -> MinMax1/1
  Subtract3/1 -> MinMax/1
  Constant6/1 -> MinMax/2
  Subtract2/1 -> Subtract3/1
  Constant2/1 -> Subtract3/2
  Constant5/1 -> Subtract2/2
  Trigonometric Function2/1 -> Gain2/1
  Divide/1 -> Divide1/1
  angle_pinc_valve (rad)/1 -> Abs/1, Trigonometric Function1/1, Scope1/1
  Gain2/1 -> Subtract1/2
  Math Function/1 -> Divide1/2
  Sqrt/1 -> Gain1/1, Scope4/1
  Abs/1 -> Trigonometric Function2/1
  Gain1/1 -> Subtract1/1
  Subtract1/1 -> Subtract2/1
  Constant3/1 -> Divide/2
  Subtract/1 -> Sqrt/1
  Divide1/1 -> Subtract/2
  Constant4/1 -> Subtract/1
  Trigonometric Function1/1 -> Math Function/1
  Constant1/1 -> Divide/1

== system MIL_pController/PLANT_MODEL/Modèle Pdc_vanne_inspi/DIV ==
  DENOM : Inport
  NUM : Inport  Port=2
  DFLT : Inport  Port=3
  Action_Else : Subsystem  TreatAsAtomicUnit=on
  Action_If : Subsystem  TreatAsAtomicUnit=on
  If : If  IfExpression=u1 ~= 0
  Merge : Merge
  RESULT : Outport
  wires:
  If/1 -> Action_If/Action
  NUM/1 -> Action_If/1(NUM)
  DENOM/1 -> Action_If/2(DENOM), If/1
  DFLT/1 -> Action_Else/1(DFLT)
  If/2 -> Action_Else/Action
  Action_If/1(RESULT) -> Merge/1
  Action_Else/1(RESULT) -> Merge/2
  Merge/1 -> RESULT/1

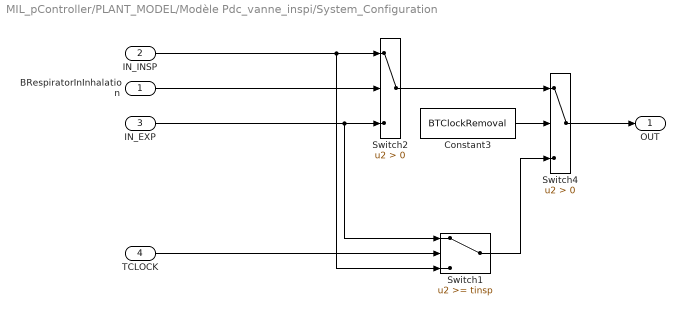
== system MIL_pController/PLANT_MODEL/Modèle Pdc_vanne_inspi/System_Configuration ==
  BRespiratorInInhalation : Inport
  IN_INSP : Inport  Port=2
  IN_EXP : Inport  Port=3
  TCLOCK : Inport  Port=4
  Constant3 : Constant  Value=BTClockRemoval
  Switch1 : Switch  Threshold=tinsp
  Switch2 : Switch  Criteria=u2 > Threshold
      settings: AttributesFormatString=%<Criteria>
  Switch4 : Switch  Criteria=u2 > Threshold
      settings: AttributesFormatString=%<Criteria>
  OUT : Outport
  wires:
  IN_EXP/1 -> Switch2/3, Switch1/1
  BRespiratorInInhalation/1 -> Switch2/2
  IN_INSP/1 -> Switch2/1, Switch1/3
  Switch4/1 -> OUT/1
  TCLOCK/1 -> Switch1/2
  Switch1/1 -> Switch4/3
  Switch2/1 -> Switch4/1
  Constant3/1 -> Switch4/2

== system MIL_pController/PLANT_MODEL/Modèle_Pdc_vanne_expi/DIV ==
  DENOM : Inport
  NUM : Inport  Port=2
  DFLT : Inport  Port=3
  Action_Else : Subsystem  TreatAsAtomicUnit=on
  Action_If : Subsystem  TreatAsAtomicUnit=on
  If : If  IfExpression=u1 ~= 0
  Merge : Merge
  RESULT : Outport
  wires:
  If/1 -> Action_If/Action
  NUM/1 -> Action_If/1(NUM)
  DENOM/1 -> Action_If/2(DENOM), If/1
  DFLT/1 -> Action_Else/1(DFLT)
  If/2 -> Action_Else/Action
  Action_If/1(RESULT) -> Merge/1
  Action_Else/1(RESULT) -> Merge/2
  Merge/1 -> RESULT/1

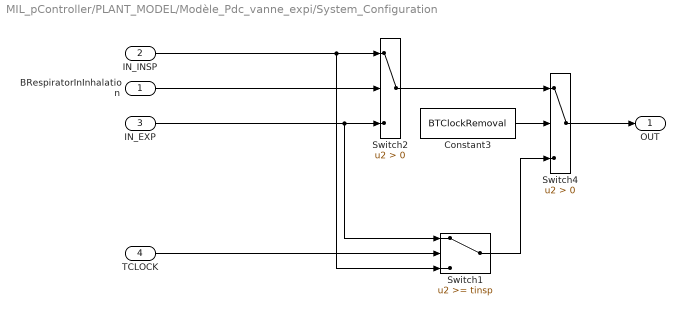
== system MIL_pController/PLANT_MODEL/Modèle_Pdc_vanne_expi/System_Configuration ==
  BRespiratorInInhalation : Inport
  IN_INSP : Inport  Port=2
  IN_EXP : Inport  Port=3
  TCLOCK : Inport  Port=4
  Constant3 : Constant  Value=BTClockRemoval
  Switch1 : Switch  Threshold=tinsp
  Switch2 : Switch  Criteria=u2 > Threshold
      settings: AttributesFormatString=%<Criteria>
  Switch4 : Switch  Criteria=u2 > Threshold
      settings: AttributesFormatString=%<Criteria>
  OUT : Outport
  wires:
  IN_EXP/1 -> Switch2/3, Switch1/1
  BRespiratorInInhalation/1 -> Switch2/2
  IN_INSP/1 -> Switch2/1, Switch1/3
  Switch4/1 -> OUT/1
  TCLOCK/1 -> Switch1/2
  Switch1/1 -> Switch4/3
  Switch2/1 -> Switch4/1
  Constant3/1 -> Switch4/2

== system MIL_pController/PLANT_MODEL/Poumon/System_Configuration ==
  BRespiratorInInhalation : Inport
  IN_EXP : Inport  Port=2
  IN_INSP : Inport  Port=3
  TCLOCK : Inport  Port=4
  Constant3 : Constant  Value=BTClockRemoval
  Switch1 : Switch  Threshold=tinsp
  Switch2 : Switch  Criteria=u2 > Threshold
      settings: AttributesFormatString=%<Criteria>
  Switch4 : Switch  Criteria=u2 > Threshold
      settings: AttributesFormatString=%<Criteria>
  OUT : Outport
  wires:
  IN_EXP/1 -> Switch2/3, Switch1/1
  BRespiratorInInhalation/1 -> Switch2/2
  IN_INSP/1 -> Switch2/1, Switch1/3
  Switch4/1 -> OUT/1
  TCLOCK/1 -> Switch1/2
  Switch1/1 -> Switch4/3
  Switch2/1 -> Switch4/1
  Constant3/1 -> Switch4/2

== system MIL_pController/PLANT_MODEL/Modèle Pdc_vanne_inspi/DIV/Action_Else ==
  DFLT : Inport
  Action Port : ActionPort  ActionType=else
  Signal Conversion : SignalConversion  OverrideOpt=off
  RESULT : Outport
  wires:
  DFLT/1 -> Signal Conversion/1
  Signal Conversion/1 -> RESULT/1

== system MIL_pController/PLANT_MODEL/Modèle Pdc_vanne_inspi/DIV/Action_If ==
  NUM : Inport
  DENOM : Inport  Port=2
  Action Port : ActionPort  ActionType=then
  Ideal gas law2 : Product  Inputs=*/
  RESULT : Outport
  wires:
  NUM/1 -> Ideal gas law2/1
  Ideal gas law2/1 -> RESULT/1
  DENOM/1 -> Ideal gas law2/2

== system MIL_pController/PLANT_MODEL/Modèle_Pdc_vanne_expi/DIV/Action_Else ==
  DFLT : Inport
  Action Port : ActionPort  ActionType=else
  Signal Conversion : SignalConversion  OverrideOpt=off
  RESULT : Outport
  wires:
  DFLT/1 -> Signal Conversion/1
  Signal Conversion/1 -> RESULT/1

== system MIL_pController/PLANT_MODEL/Modèle_Pdc_vanne_expi/DIV/Action_If ==
  NUM : Inport
  DENOM : Inport  Port=2
  Action Port : ActionPort  ActionType=then
  Ideal gas law2 : Product  Inputs=*/
  RESULT : Outport
  wires:
  NUM/1 -> Ideal gas law2/1
  Ideal gas law2/1 -> RESULT/1
  DENOM/1 -> Ideal gas law2/2

== matlab function MIL_pController/PLANT_MODEL/Poumon/MATLAB Function1 ==
  data: u input; y output; v input; w input; y2 output
function [y,y2] = fcn(u,v,w)
vec=roots([-u v w]);
if vec(1,1)>0
    y = real(vec(1,1));
    y2= real(vec(2,1));
else
y = real(vec(2,1));
y2=real(vec(1,1));
end;

== matlab function MIL_pController/PLANT_MODEL/Poumon/MATLAB Function ==
  data: u input; y output; v input; w input; y2 output
function [y,y2] = fcn(u,v,w)
vec=roots([u v w]);
if vec(1,1)>0
    y = real(vec(1,1));
    y2= real(vec(2,1));
else
y = real(vec(2,1));
y2=real(vec(1,1));
end;
